simulink model "acc_lk_controller"  (R2017a)
settings: Solver=VariableStepAuto  StartTime=0.0  StopTime=10.0  RelTol=1e-3
settings Model: Creator=laptopuser  LastModifiedBy=User

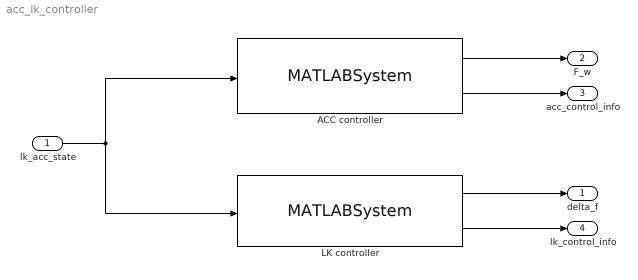
== system acc_lk_controller ==
  lk_acc_state : Inport  OutDataTypeStr=Bus: LKACCBus
  ACC controller : MATLABSystem  System=acc_pcis_controller  M=1800  f0bar=74.63  f1bar=40.59  vl=26/3.6  H_x=diag([1 0.001])  f_x=[-28/3.6;0]  H_u=0.0001  f_u=0  sol_opts=struct( 'DataType', 'double', 'MaxIter', 200, 'FeasibilityTol', 1e-6, 'IntegrityChecks', true )  SimulateUsing=Code generation
      mask Type: acc_pcis_controller
      mask Display:
      | disp('acc_pcis_controller');
      | port_label('input',1,'lk_acc_state');
      | port_label('output',1,'F_w');
      | port_label('output',2,'control_info');
  LK controller : MATLABSystem  System=lk_pcis_controller  M=1800  lf=1.2  lr=1.650  Caf=140000  Car=120000  Iz=3270.0  H_x=diag([1 0 0.5 0])  f_x=[0;0;0;0]  H_u=0.25  f_u=0  sol_opts=struct( 'DataType', 'double', 'MaxIter', 200, 'FeasibilityTol', 1e-6, 'IntegrityChecks', true )  SimulateUsing=Code generation
      mask Type: lk_pcis_controller
      mask Display:
      | disp('lk_pcis_controller');
      | port_label('input',1,'lk_state');
      | port_label('output',1,'delta_f');
      | port_label('output',2,'control_info');
  delta_f : Outport
  F_w : Outport  Port=2
  acc_control_info : Outport  Port=3  OutDataTypeStr=Bus: ControlInfoBus
  lk_control_info : Outport  Port=4  OutDataTypeStr=Bus: ControlInfoBus
  wires:
  LK controller/2 -> lk_control_info/1
  ACC controller/2 -> acc_control_info/1
  lk_acc_state/1 -> ACC controller/1, LK controller/1
  ACC controller/1 -> F_w/1
  LK controller/1 -> delta_f/1
